simulink model "RockySimulink"  (R2024b)
settings: Solver=VariableStepAuto  StartTime=0.0  StopTime=7  RelTol=1e-3
values from neighbouring files (symbols this model uses):
  a = 23.2135    [RockySimulinkVariables.m]    (also in Rocky_5_closed_loop_poles.m; Rocky_closed_loop_poles_23.m; calibration.m = model.a)
  b = 0.003    [RockySimulinkVariables.m]    (also in Rocky_5_closed_loop_poles.m; Rocky_closed_loop_poles_23.m = 0.0025; regress_underdamped_response.m = (M'*M)\(M'*x_data))
  Ci = 0.14    [RockySimulinkVariables.m]
  Ji = 0.13    [RockySimulinkVariables.m]
  Jp = 0.12    [RockySimulinkVariables.m]
  Ki = 269020    [RockySimulinkVariables.m]    (also in Rocky_closed_loop_poles_23.m = (ell_eff/(alpha*beta_eff))*(alpha^3/27 + alpha*omega_n^2))
  Kp = 57744    [RockySimulinkVariables.m]    (also in Rocky_closed_loop_poles_23.m = (ell_eff/(alpha*beta_eff))*(alpha^2/3 + omega_n^2))
  l = 0.4873    [RockySimulinkVariables.m]    (also in Rocky_5_closed_loop_poles.m; Rocky_closed_loop_poles_23.m = 0.5588)
  omegan = 4.4869    [RockySimulinkVariables.m]
settings Model: Creator=ltrepte  LastModifiedBy=ltrepte

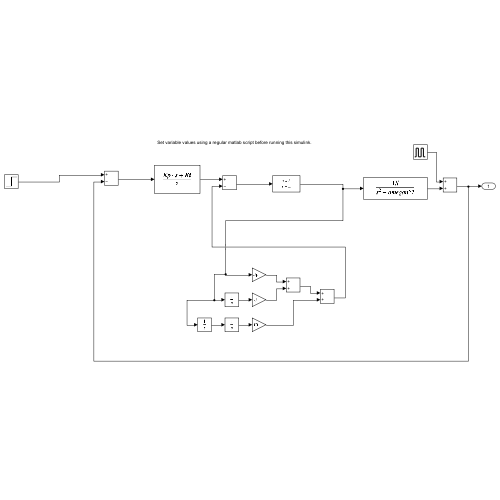
[thumbnail: Simulink's stored preview of the top-level diagram]
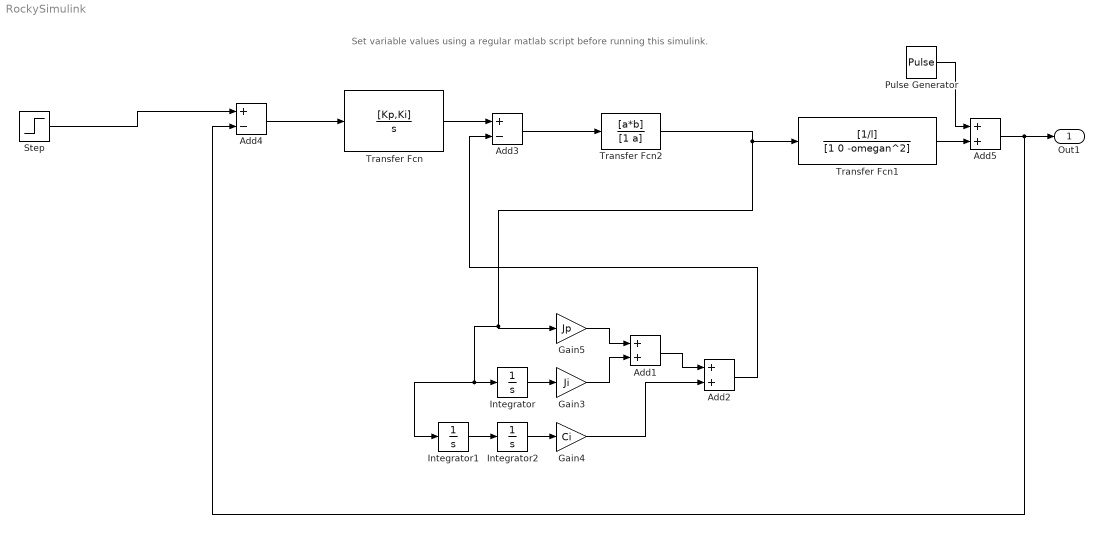
== system RockySimulink ==
  note: Set variable values using a regular matlab script before running this simulink.
  Add1 : Sum
  Add2 : Sum
  Add3 : Sum  Inputs=+-
  Add4 : Sum  Inputs=+-
  Add5 : Sum
  Gain3 : Gain  Gain=Ji
  Gain4 : Gain  Gain=Ci
  Gain5 : Gain  Gain=Jp
  Integrator : Integrator
  Integrator1 : Integrator
  Integrator2 : Integrator
  Pulse Generator : DiscretePulseGenerator  PulseType=Time based  Period=10  PulseWidth=3  PhaseDelay=5
  Step : Step  Time=0  After=0  SampleTime=0
  Transfer Fcn : TransferFcn  Numerator=[Kp,Ki]  Denominator=[1,0]
  Transfer Fcn1 : TransferFcn  Numerator=[1/l]  Denominator=[1 0 -omegan^2]
  Transfer Fcn2 : TransferFcn  Numerator=[a*b]  Denominator=[1 a]
  Out1 : Outport
  wires:
  Transfer Fcn2/1 -> Integrator/1, Integrator1/1, Gain5/1, Transfer Fcn1/1
  Integrator1/1 -> Integrator2/1
  Integrator2/1 -> Gain4/1
  Integrator/1 -> Gain3/1
  Gain4/1 -> Add2/2
  Gain3/1 -> Add1/2
  Gain5/1 -> Add1/1
  Add1/1 -> Add2/1
  Add2/1 -> Add3/2
  Transfer Fcn/1 -> Add3/1
  Add4/1 -> Transfer Fcn/1
  Transfer Fcn1/1 -> Add5/2
  Pulse Generator/1 -> Add5/1
  Step/1 -> Add4/1
  Add5/1 -> Add4/2, Out1/1
  Add3/1 -> Transfer Fcn2/1
